simulink model "Simulation_Block_Diagram_PowerElectronics"  (R2015b)
settings: Solver=ode23tb  StartTime=0.0  StopTime=1  FixedStep=1e-7  MaxStep=1e-5  MinStep=1e-20  RelTol=1e-3  AbsTol=1e-3
undefined symbols (not defined in the file): C, K_d, K_q, L, lambda, Ld, Lq, P, R, rs, V_batt, w_r
libraries: simulink x2
settings Model: Creator=ahmedm  LastModifiedBy=Kane Chew
settings SolverCC: ZeroCrossControl=EnableAll  ZeroCrossAlgorithm=Adaptive
settings DataIOCC: SaveFormat=Array  SignalLoggingSaveFormat=ModelDataLogs
settings OptimizationCC: ExpressionDepthLimit=2147483647
settings DebuggingCC: UnderspecifiedInitializationDetection=Classic  MergeDetectMultiDrivingBlocksExec=none  SolverPrmCheckMsg=warning  FcnCallInpInsideContextMsg=EnableAllAsWarning  StateNameClashWarn=warning
settings HardwareCC: ProdBitPerPointer=32  ProdLargestAtomicFloat=None  ProdIntDivRoundTo=Undefined  ProdEndianess=Unspecified  ProdWordSize=32  ProdHWDeviceType=32-bit Generic
settings GRTTargetCC: GeneratePreprocessorConditionals=Disable all  CombineOutputUpdateFcns=off  GRTInterface=on
settings ConfigComp: CovModelRefEnable=Off

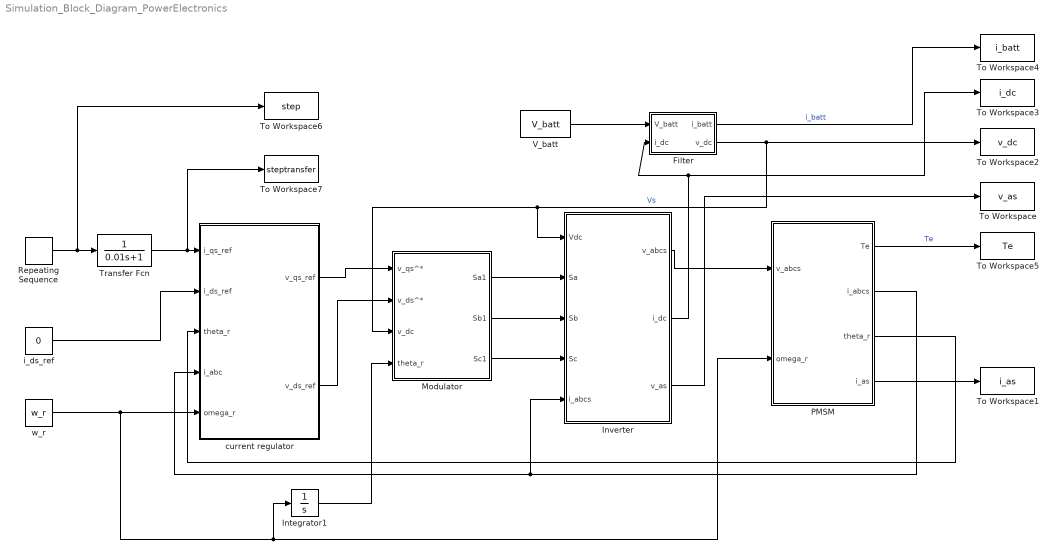
== system Simulation_Block_Diagram_PowerElectronics ==
  Filter : Subsystem
  Integrator1 : Integrator
  Inverter : Subsystem
  Modulator : Subsystem
  PMSM : Subsystem
  Repeating Sequence : simulink/Sources/Repeating Sequence  rep_seq_t=[0 0.2 0.201 0.5 0.501 0.8 0.801 1]  rep_seq_y=[0 0 209 209 -209 -209 0 0]
  To Workspace : ToWorkspace  VariableName=v_as  SaveFormat=Timeseries  SampleTime=-1
  To Workspace1 : ToWorkspace  VariableName=i_as  SaveFormat=Timeseries  SampleTime=-1
  To Workspace2 : ToWorkspace  VariableName=v_dc  SaveFormat=Timeseries  SampleTime=-1
  To Workspace3 : ToWorkspace  VariableName=i_dc  SaveFormat=Timeseries  SampleTime=-1
  To Workspace4 : ToWorkspace  VariableName=i_batt  SaveFormat=Timeseries  SampleTime=-1
  To Workspace5 : ToWorkspace  VariableName=Te  SaveFormat=Timeseries  SampleTime=-1
  To Workspace6 : ToWorkspace  VariableName=step  SaveFormat=Timeseries  SampleTime=-1
  To Workspace7 : ToWorkspace  VariableName=steptransfer  SaveFormat=Timeseries  SampleTime=-1
  Transfer Fcn : TransferFcn  Denominator=[0.01 1]
  V_batt : Constant  Value=V_batt
  current regulator : Subsystem
  i_ds_ref : Constant  Value=0
  w_r : Constant  Value=w_r
  wires:
  w_r/1 -> PMSM/2(omega_r), Integrator1/1, current regulator/5(omega_r)
  PMSM/2(i_abcs) -> Inverter/5(i_abcs), current regulator/4(i_abc)
  PMSM/3(theta_r) -> current regulator/3(theta_r)
  Inverter/2(i_dc) -> To Workspace3/1, Filter/2(i_dc)
  Inverter/1(v_abcs) -> PMSM/1(v_abcs)
  Modulator/1(Sa1) -> Inverter/2(Sa)
  Modulator/2(Sb1) -> Inverter/3(Sb)
  Modulator/3(Sc1) -> Inverter/4(Sc)
  current regulator/2(v_ds_ref) -> Modulator/2(v_ds^*)
  Filter/2(v_dc) -> To Workspace2/1, Modulator/3(v_dc), Inverter/1(Vdc)  "Vs"
  Integrator1/1 -> Modulator/4(theta_r)
  PMSM/1(Te) -> To Workspace5/1  "Te"
  i_ds_ref/1 -> current regulator/2(i_ds_ref)
  V_batt/1 -> Filter/1(V_batt)
  current regulator/1(v_qs_ref) -> Modulator/1(v_qs^*)
  Filter/1(i_batt) -> To Workspace4/1  "i_batt"
  Inverter/3(v_as) -> To Workspace/1
  Repeating Sequence/1 -> To Workspace6/1, Transfer Fcn/1
  Transfer Fcn/1 -> To Workspace7/1, current regulator/1(i_qs_ref)
  PMSM/4(i_as) -> To Workspace1/1

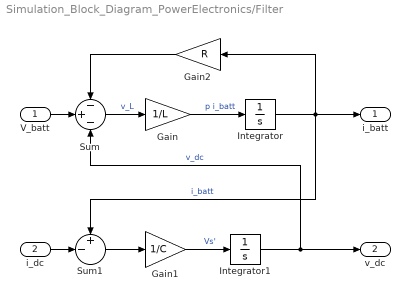
== system Simulation_Block_Diagram_PowerElectronics/Filter ==
  V_batt : Inport
  i_dc : Inport  Port=2
  Gain : Gain  Gain=1/L
  Gain1 : Gain  Gain=1/C
  Gain2 : Gain  Gain=R
  Integrator : Integrator
  Integrator1 : Integrator  InitialCondition=V_batt
  Sum : Sum  Inputs=-+-
  Sum1 : Sum  Inputs=+-|
  i_batt : Outport
  v_dc : Outport  Port=2
  wires:
  Sum/1 -> Gain/1  "v_L"
  Gain/1 -> Integrator/1  "p i_batt"
  Integrator/1 -> Gain2/1, i_batt/1, Sum1/1  "i_batt"
  i_dc/1 -> Sum1/2
  Sum1/1 -> Gain1/1
  Integrator1/1 -> v_dc/1, Sum/3  "v_dc"
  Gain1/1 -> Integrator1/1  "Vs'"
  V_batt/1 -> Sum/2
  Gain2/1 -> Sum/1

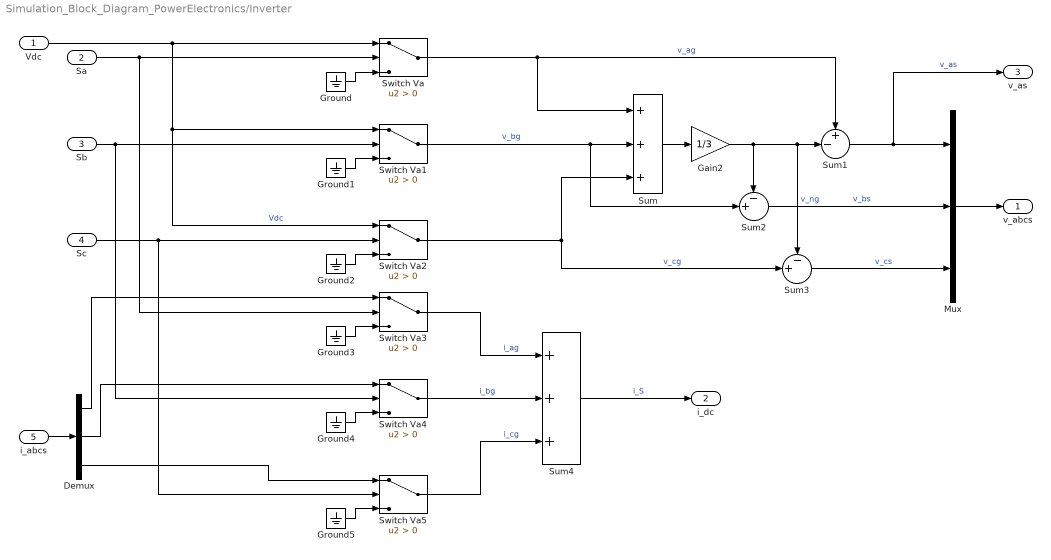
== system Simulation_Block_Diagram_PowerElectronics/Inverter ==
  Vdc : Inport
  Sa : Inport  Port=2
  Sb : Inport  Port=3
  Sc : Inport  Port=4
  i_abcs : Inport  Port=5
  Demux : Demux  Outputs=3
  Gain2 : Gain  Gain=1/3
  Ground{,1..5} (6 alike) : Ground
  Mux : Mux  Inputs=3
  Sum : Sum  Inputs=+++
  Sum1 : Sum  Inputs=+-|
  Sum2 : Sum  Inputs=-+|
  Sum3 : Sum  Inputs=-+|
  Sum4 : Sum  Inputs=+++
  Switch Va{,1..5} (6 alike) : Switch  Criteria=u2 > Threshold
  v_abcs : Outport
  i_dc : Outport  Port=2
  v_as : Outport  Port=3
  wires:
  Ground/1 -> Switch Va/3
  Ground1/1 -> Switch Va1/3
  Ground2/1 -> Switch Va2/3
  Vdc/1 -> Switch Va1/1, Switch Va2/1, Switch Va/1  "Vdc"
  Sa/1 -> Switch Va/2, Switch Va3/2
  Sb/1 -> Switch Va1/2, Switch Va4/2
  Sc/1 -> Switch Va2/2, Switch Va5/2
  Switch Va/1 -> Sum/1, Sum1/1  "v_ag"
  Switch Va1/1 -> Sum/2, Sum2/2  "v_bg"
  Switch Va2/1 -> Sum/3, Sum3/2  "v_cg"
  Sum/1 -> Gain2/1
  Gain2/1 -> Sum2/1, Sum1/2, Sum3/1  "v_ng"
  Ground3/1 -> Switch Va3/3
  Ground4/1 -> Switch Va4/3
  Ground5/1 -> Switch Va5/3
  Switch Va3/1 -> Sum4/1  "i_ag"
  Switch Va4/1 -> Sum4/2  "i_bg"
  Switch Va5/1 -> Sum4/3  "i_cg"
  Sum2/1 -> Mux/2  "v_bs"
  Sum3/1 -> Mux/3  "v_cs"
  Demux/2 -> Switch Va4/1
  Sum4/1 -> i_dc/1  "i_S"
  Demux/3 -> Switch Va5/1
  i_abcs/1 -> Demux/1
  Demux/1 -> Switch Va3/1
  Mux/1 -> v_abcs/1
  Sum1/1 -> v_as/1, Mux/1  "v_as"

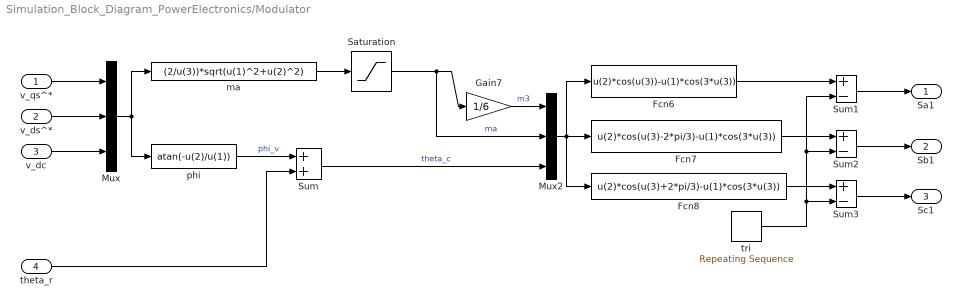
== system Simulation_Block_Diagram_PowerElectronics/Modulator ==
  v_qs^* : Inport
  v_ds^* : Inport  Port=2
  v_dc : Inport  Port=3
  theta_r : Inport  Port=4
  Fcn6 : Fcn  Expr=u(2)*cos(u(3))-u(1)*cos(3*u(3))
  Fcn7 : Fcn  Expr=u(2)*cos(u(3)-2*pi/3)-u(1)*cos(3*u(3))
  Fcn8 : Fcn  Expr=u(2)*cos(u(3)+2*pi/3)-u(1)*cos(3*u(3))
  Gain7 : Gain  Gain=1/6
  Mux : Mux  Inputs=3
  Mux2 : Mux  Inputs=3
  Saturation : Saturate  UpperLimit=1.15  LowerLimit=0
  Sum : Sum
  Sum1 : Sum  Inputs=+-
  Sum2 : Sum  Inputs=+-
  Sum3 : Sum  Inputs=+-
  ma : Fcn  Expr=(2/u(3))*sqrt(u(1)^2+u(2)^2)
  phi : Fcn  Expr=atan(-u(2)/u(1))
  tri : simulink/Sources/Repeating Sequence  rep_seq_t=[0 1/40000 1/20000 3/40000 1/10000]  rep_seq_y=[0 1 0 -1 0]
  Sa1 : Outport
  Sb1 : Outport  Port=2
  Sc1 : Outport  Port=3
  wires:
  tri/1 -> Sum3/2, Sum2/2, Sum1/2
  Sum1/1 -> Sa1/1
  Sum2/1 -> Sb1/1
  Sum3/1 -> Sc1/1
  v_qs^*/1 -> Mux/1
  v_ds^*/1 -> Mux/2
  v_dc/1 -> Mux/3
  Mux/1 -> ma/1, phi/1
  phi/1 -> Sum/1  "phi_v"
  Sum/1 -> Mux2/3  "theta_c"
  Mux2/1 -> Fcn6/1, Fcn7/1, Fcn8/1
  Gain7/1 -> Mux2/1  "m3"
  Fcn6/1 -> Sum1/1
  Fcn7/1 -> Sum2/1
  Fcn8/1 -> Sum3/1
  ma/1 -> Saturation/1
  Saturation/1 -> Gain7/1, Mux2/2  "ma"
  theta_r/1 -> Sum/2

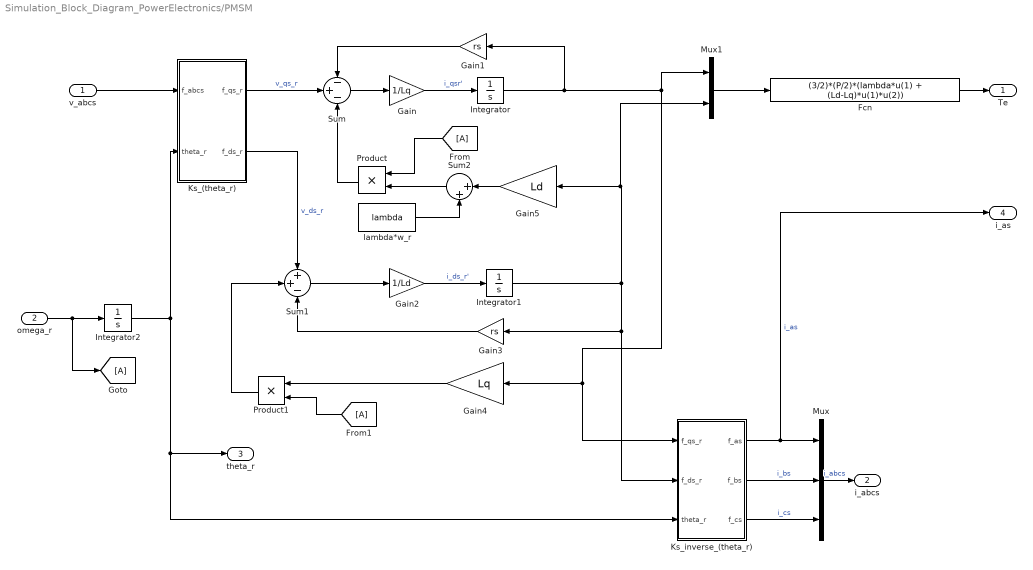
== system Simulation_Block_Diagram_PowerElectronics/PMSM ==
  v_abcs : Inport
  omega_r : Inport  Port=2
  Fcn : Fcn  Expr=(3/2)*(P/2)*(lambda*u(1) + (Ld-Lq)*u(1)*u(2))
  Gain : Gain  Gain=1/Lq
  Gain1 : Gain  Gain=rs
  Gain2 : Gain  Gain=1/Ld
  Gain3 : Gain  Gain=rs
  Gain4 : Gain  Gain=Lq
  Gain5 : Gain  Gain=Ld
  Integrator : Integrator
  Integrator1 : Integrator
  Integrator2 : Integrator
  Ks_(theta_r) : Subsystem
  Ks_inverse_(theta_r) : Subsystem
  Mux : Mux  Inputs=3
  Mux1 : Mux  Inputs=2
  Product : Product
  Product1 : Product
  Sum : Sum  Inputs=-+-
  Sum1 : Sum  Inputs=++-
  Sum2 : Sum  Inputs=|++
  lambda*w_r : Constant  Value=lambda
  Te : Outport
  i_abcs : Outport  Port=2
  theta_r : Outport  Port=3
  i_as : Outport  Port=4
  wires:
  Ks_(theta_r)/2(f_ds_r) -> Sum1/1  "v_ds_r"
  Ks_(theta_r)/1(f_qs_r) -> Sum/2  "v_qs_r"
  Sum/1 -> Gain/1
  Gain/1 -> Integrator/1  "i_qsr'"
  Integrator/1 -> Mux1/1, Gain4/1, Ks_inverse_(theta_r)/1(f_qs_r), Gain1/1
  Sum1/1 -> Gain2/1
  Gain2/1 -> Integrator1/1  "i_ds_r'"
  Integrator1/1 -> Mux1/2, Gain5/1, Gain3/1, Ks_inverse_(theta_r)/2(f_ds_r)
  Gain3/1 -> Sum1/3
  Integrator2/1 -> Ks_(theta_r)/2(theta_r), Ks_inverse_(theta_r)/3(theta_r), theta_r/1
  Ks_inverse_(theta_r)/1(f_as) -> i_as/1, Mux/1  "i_as"
  Ks_inverse_(theta_r)/2(f_bs) -> Mux/2  "i_bs"
  Ks_inverse_(theta_r)/3(f_cs) -> Mux/3  "i_cs"
  Fcn/1 -> Te/1
  Mux/1 -> i_abcs/1  "i_abcs"
  v_abcs/1 -> Ks_(theta_r)/1(f_abcs)
  omega_r/1 -> [A], Integrator2/1
  Gain5/1 -> Sum2/1
  lambda*w_r/1 -> Sum2/2
  Sum2/1 -> Product/2
  Gain1/1 -> Sum/1
  Product/1 -> Sum/3
  [A] -> Product/1
  Gain4/1 -> Product1/1
  Product1/1 -> Sum1/2
  [A] -> Product1/2
  Mux1/1 -> Fcn/1

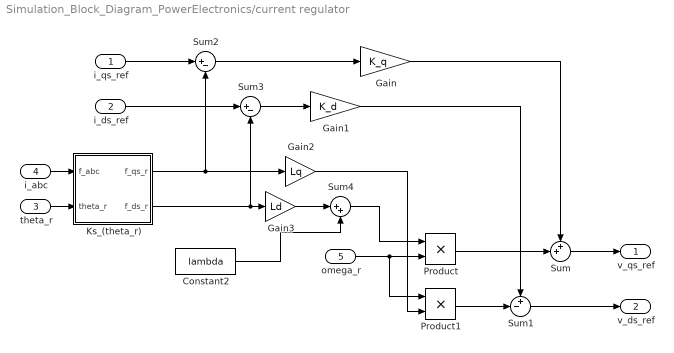
== system Simulation_Block_Diagram_PowerElectronics/current regulator ==
  i_qs_ref : Inport
  i_ds_ref : Inport  Port=2
  theta_r : Inport  Port=3
  i_abc : Inport  Port=4
  omega_r : Inport  Port=5
  Constant2 : Constant  Value=lambda
  Gain : Gain  Gain=K_q
  Gain1 : Gain  Gain=K_d
  Gain2 : Gain  Gain=Lq
  Gain3 : Gain  Gain=Ld
  Ks_(theta_r) : Subsystem
  Product : Product
  Product1 : Product
  Sum : Sum  Inputs=++|
  Sum1 : Sum  Inputs=+-|
  Sum2 : Sum  Inputs=|+-
  Sum3 : Sum  Inputs=|+-
  Sum4 : Sum  Inputs=|++
  v_qs_ref : Outport
  v_ds_ref : Outport  Port=2
  wires:
  theta_r/1 -> Ks_(theta_r)/2(theta_r)
  Product/1 -> Sum/2
  omega_r/1 -> Product1/1, Product/2
  Sum/1 -> v_qs_ref/1
  Product1/1 -> Sum1/2
  Sum1/1 -> v_ds_ref/1
  Sum2/1 -> Gain/1
  Sum3/1 -> Gain1/1
  Gain/1 -> Sum/1
  Gain1/1 -> Sum1/1
  i_ds_ref/1 -> Sum3/1
  i_qs_ref/1 -> Sum2/1
  i_abc/1 -> Ks_(theta_r)/1(f_abc)
  Ks_(theta_r)/1(f_qs_r) -> Gain2/1, Sum2/2
  Ks_(theta_r)/2(f_ds_r) -> Sum3/2, Gain3/1
  Gain2/1 -> Product1/2
  Gain3/1 -> Sum4/1
  Sum4/1 -> Product/1
  Constant2/1 -> Sum4/2

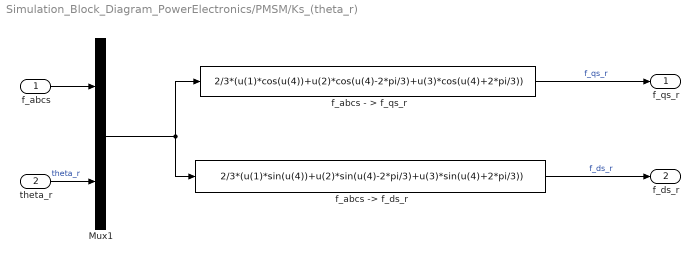
== system Simulation_Block_Diagram_PowerElectronics/PMSM/Ks_(theta_r) ==
  f_abcs : Inport
  theta_r : Inport  Port=2
  Mux1 : Mux  Inputs=2
  f_abcs - > f_qs_r : Fcn  Expr=2/3*(u(1)*cos(u(4))+u(2)*cos(u(4)-2*pi/3)+u(3)*cos(u(4)+2*pi/3))
  "f_abcs -> f_ds_r" : Fcn  Expr=2/3*(u(1)*sin(u(4))+u(2)*sin(u(4)-2*pi/3)+u(3)*sin(u(4)+2*pi/3))
  f_qs_r : Outport
  f_ds_r : Outport  Port=2
  wires:
  "f_abcs -> f_ds_r"/1 -> f_ds_r/1  "f_ds_r"
  f_abcs/1 -> Mux1/1
  f_abcs - > f_qs_r/1 -> f_qs_r/1  "f_qs_r"
  Mux1/1 -> "f_abcs -> f_ds_r"/1, f_abcs - > f_qs_r/1
  theta_r/1 -> Mux1/2  "theta_r"

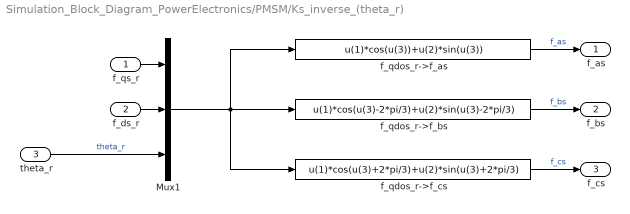
== system Simulation_Block_Diagram_PowerElectronics/PMSM/Ks_inverse_(theta_r) ==
  f_qs_r : Inport
  f_ds_r : Inport  Port=2
  theta_r : Inport  Port=3
  Mux1 : Mux  Inputs=3
  f_qdos_r->f_as : Fcn  Expr=u(1)*cos(u(3))+u(2)*sin(u(3))
  f_qdos_r->f_bs : Fcn  Expr=u(1)*cos(u(3)-2*pi/3)+u(2)*sin(u(3)-2*pi/3)
  f_qdos_r->f_cs : Fcn  Expr=u(1)*cos(u(3)+2*pi/3)+u(2)*sin(u(3)+2*pi/3)
  f_as : Outport
  f_bs : Outport  Port=2
  f_cs : Outport  Port=3
  wires:
  theta_r/1 -> Mux1/3  "theta_r"
  Mux1/1 -> f_qdos_r->f_as/1, f_qdos_r->f_bs/1, f_qdos_r->f_cs/1
  f_qdos_r->f_as/1 -> f_as/1  "f_as"
  f_qs_r/1 -> Mux1/1
  f_ds_r/1 -> Mux1/2
  f_qdos_r->f_bs/1 -> f_bs/1  "f_bs"
  f_qdos_r->f_cs/1 -> f_cs/1  "f_cs"

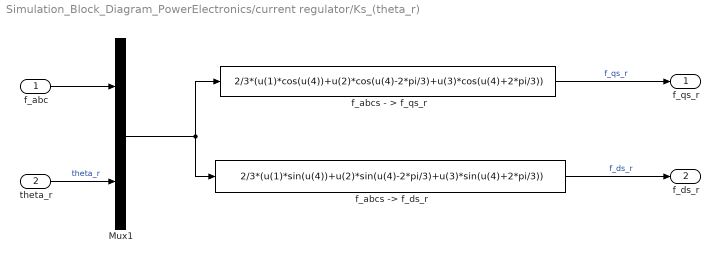
== system Simulation_Block_Diagram_PowerElectronics/current regulator/Ks_(theta_r) ==
  f_abc : Inport
  theta_r : Inport  Port=2
  Mux1 : Mux  Inputs=2
  f_abcs - > f_qs_r : Fcn  Expr=2/3*(u(1)*cos(u(4))+u(2)*cos(u(4)-2*pi/3)+u(3)*cos(u(4)+2*pi/3))
  "f_abcs -> f_ds_r" : Fcn  Expr=2/3*(u(1)*sin(u(4))+u(2)*sin(u(4)-2*pi/3)+u(3)*sin(u(4)+2*pi/3))
  f_qs_r : Outport
  f_ds_r : Outport  Port=2
  wires:
  "f_abcs -> f_ds_r"/1 -> f_ds_r/1  "f_ds_r"
  f_abc/1 -> Mux1/1
  f_abcs - > f_qs_r/1 -> f_qs_r/1  "f_qs_r"
  Mux1/1 -> "f_abcs -> f_ds_r"/1, f_abcs - > f_qs_r/1
  theta_r/1 -> Mux1/2  "theta_r"
